simulink model "07.demux"  (R2019b)
settings: Solver=FixedStepAuto  StartTime=0.0  StopTime=inf  FixedStep=1  MaxStep=1  RelTol=1e-3
libraries: simulink x2
settings Model: Creator=MARAT  LastModifiedBy=Marat
settings SFSimCC: CustomCodeUndefinedFunction=UseInterfaceOnly

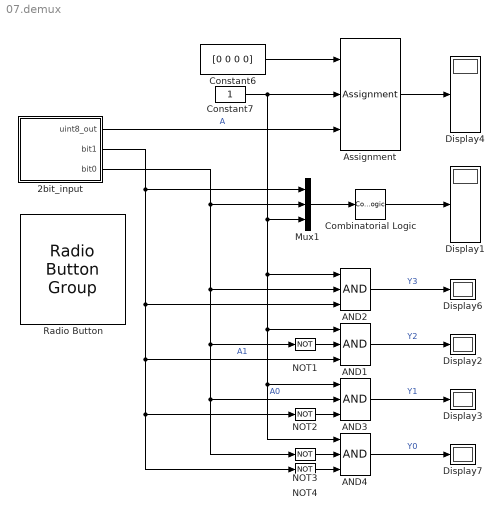
== system 07.demux ==
  2bit_input : Subsystem
      mask Display: image('D:\Work\DS_in_SL\funpics\2bit.jpg'); % Use "Edit Image" on toolstrip to change.
  AND{1..4} (4 alike) : Logic  Inputs=3  IconShape=distinctive  AllPortsSameDT=off  OutDataTypeStr=boolean
  Assignment : Assignment  IndexMode=Zero-based  DiagnosticForDimensions=Warning  IndexOptions=Index vector (port)  Indices=1  OutputSizes=1
  Combinatorial Logic : CombinatorialLogic  TruthTable=[0 0 0 0; 0 0 0 1; 0 0 0 0; 0 0 1 0; 0 0 0 0; 0 1 0 0; 0 0 0 0; 1 0 0 0]
  Constant6 : Constant  Value=[0 0 0 0]  OutDataTypeStr=boolean
  Constant7 : Constant  OutDataTypeStr=boolean
  Display{1..4,6..7} (6 alike) : Display
  Mux1 : Mux  Inputs=3
  NOT{1..4} (4 alike) : Logic  Operator=NOT  IconShape=distinctive  AllPortsSameDT=off  OutDataTypeStr=boolean
  Radio Button : RadioButtonGroup  SelectedLabel=0
      settings: Values={{'0', '1', '2', '3'}, [0 1 2 3]}
  wires:
  Combinatorial Logic/1 -> Display1/1
  Constant6/1 -> Assignment/1
  Assignment/1 -> Display4/1
  Mux1/1 -> Combinatorial Logic/1
  Constant7/1 -> Assignment/2, AND4/1, AND3/1, AND1/1, AND2/1, Mux1/3
  AND2/1 -> Display6/1  "Y3"
  NOT1/1 -> AND1/2
  NOT2/1 -> AND3/3
  AND1/1 -> Display2/1  "Y2"
  AND3/1 -> Display3/1  "Y1"
  AND4/1 -> Display7/1  "Y0"
  NOT3/1 -> AND4/2
  NOT4/1 -> AND4/3
  2bit_input/3(bit0) -> NOT3/1, AND3/2, NOT1/1, AND2/2, Mux1/2  "A0"
  2bit_input/2(bit1) -> NOT4/1, NOT2/1, AND1/3, AND2/3, Mux1/1  "A1"
  2bit_input/1(uint8_out) -> Assignment/3  "A"

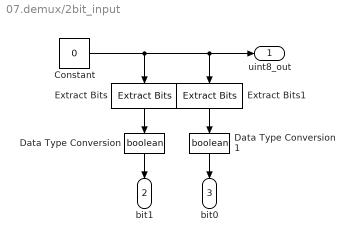
== system 07.demux/2bit_input ==
  Constant : Constant  Value=0  OutMin=0  OutMax=3  OutDataTypeStr=uint8
  Data Type Conversion : DataTypeConversion  OutDataTypeStr=boolean
  Data Type Conversion1 : DataTypeConversion  OutDataTypeStr=boolean
  Extract Bits : simulink/Logic and Bit Operations/Extract Bits  bitsToExtract=Range of bits  numBits=8  bitIdxRange=1  outScalingMode=Treat bit field as an integer
      settings: SourceProductName=Simulink
  Extract Bits1 : simulink/Logic and Bit Operations/Extract Bits  bitsToExtract=Range of bits  numBits=8  bitIdxRange=0  outScalingMode=Treat bit field as an integer
      settings: SourceProductName=Simulink
  uint8_out : Outport
  bit1 : Outport  Port=2
  bit0 : Outport  Port=3
  wires:
  Constant/1 -> uint8_out/1, Extract Bits1/1, Extract Bits/1
  Extract Bits/1 -> Data Type Conversion/1
  Data Type Conversion1/1 -> bit0/1
  Extract Bits1/1 -> Data Type Conversion1/1
  Data Type Conversion/1 -> bit1/1
